simulink model "MIL_ASW"  (R2019b)
settings: Solver=FixedStepDiscrete  StartTime=0.0  StopTime=2  FixedStep=0.001  RelTol=1e-3  EnableMultiTasking=on
model workspace (MAT data in the model file):
  AccPedlCanVal : Simulink.Signal (value not decoded)
  AccPedlVal : Simulink.Signal (value not decoded)
  BrkPedlCanVal : Simulink.Signal (value not decoded)
  BrkPedlVal : Simulink.Signal (value not decoded)
  Cal1 : Simulink.Parameter (value not decoded)
  Cal10 : Simulink.Parameter (value not decoded)
  Cal11 : Simulink.Parameter (value not decoded)
  Cal12 : Simulink.Parameter (value not decoded)
  Cal2 : Simulink.Parameter (value not decoded)
  Cal3 : Simulink.Parameter (value not decoded)
  Cal4 : Simulink.Parameter (value not decoded)
  Cal5 : Simulink.Parameter (value not decoded)
  Cal6 : Simulink.Parameter (value not decoded)
  Cal7 : Simulink.Parameter (value not decoded)
  Cal8 : Simulink.Parameter (value not decoded)
  Cal9 : Simulink.Parameter (value not decoded)
  Clu1Act : Simulink.Signal (value not decoded)
  Clu1PTar : Simulink.Signal (value not decoded)
  Clu1Req : Simulink.Signal (value not decoded)
  Clu1TqTar : Simulink.Signal (value not decoded)
  Clu2Act : Simulink.Signal (value not decoded)
  Clu2PTar : Simulink.Signal (value not decoded)
  Clu2Req : Simulink.Signal (value not decoded)
  Clu2TqTar : Simulink.Signal (value not decoded)
  CluKissPtPLnch : Simulink.Parameter (value not decoded)
  CluOilTRawVal : Simulink.Signal (value not decoded)
  CluOilTVal : Simulink.Signal (value not decoded)
  CluOpenTqRatMax : Simulink.Parameter (value not decoded)
  CluPMap : Simulink.Parameter (value not decoded)
  CluPMax : Simulink.Parameter (value not decoded)
  CluPMaxGear1 : Simulink.Parameter (value not decoded)
  CluPMaxGear2 : Simulink.Parameter (value not decoded)
  CluPMaxGear3 : Simulink.Parameter (value not decoded)
  CluPMaxGear4 : Simulink.Parameter (value not decoded)
  CluPMaxGear5 : Simulink.Parameter (value not decoded)
  CluPMaxGear6 : Simulink.Parameter (value not decoded)
  CluPMaxGearR : Simulink.Parameter (value not decoded)
  CluPMin : Simulink.Parameter (value not decoded)
  CluPosnMax : Simulink.Parameter (value not decoded)
  CluSoln1IRawVal : Simulink.Signal (value not decoded)
  CluSoln1IReq : Simulink.Signal (value not decoded)
  CluSoln1IReqFlg : Simulink.Signal (value not decoded)
  CluSoln1IVal : Simulink.Signal (value not decoded)
  CluSoln1LineI : Simulink.Parameter (value not decoded)
  CluSoln1LineP : Simulink.Parameter (value not decoded)
  CluSoln1Pwm : Simulink.Signal (value not decoded)
  CluSoln2IRawVal : Simulink.Signal (value not decoded)
  CluSoln2IReq : Simulink.Signal (value not decoded)
  CluSoln2IReqFlg : Simulink.Signal (value not decoded)
  CluSoln2IVal : Simulink.Signal (value not decoded)
  CluSoln2LineI : Simulink.Parameter (value not decoded)
  CluSoln2LineP : Simulink.Parameter (value not decoded)
  CluSoln2Pwm : Simulink.Signal (value not decoded)
  CluTqMap : Simulink.Parameter (value not decoded)
  CrnkSpdRawVal : Simulink.Signal (value not decoded)
  CrnkSpdVal : Simulink.Signal (value not decoded)
  Drive_Intensity_Fuzzy : object (value not decoded)
  DrvIntenFzzy : Simulink.LookupTable (value not decoded)
  EngNIdle : Simulink.Parameter (value not decoded)
  EngNIdleMin : Simulink.Parameter (value not decoded)
  EngSpdCanVal : Simulink.Signal (value not decoded)
  EngThrCanVal : Simulink.Signal (value not decoded)
  EngTqAdd : Simulink.Parameter (value not decoded)
  EngTqCanVal : Simulink.Signal (value not decoded)
  EngTqIntvFlg : Simulink.Signal (value not decoded)
  EngTqIntvRat : Simulink.Signal (value not decoded)
  EngTqMapExtChartc : Simulink.Parameter (value not decoded)
  EngTqMapSpdIndx : Simulink.Parameter (value not decoded)
  EngTqMapThrtIndx : Simulink.Parameter (value not decoded)
  EngTqMapTqMax : Simulink.Parameter (value not decoded)
  EngTqMaxNorm : Simulink.Parameter (value not decoded)
  EngTqRef : Simulink.Parameter (value not decoded)
  EvenCluPRawVal : Simulink.Signal (value not decoded)
  EvenCluPVal : Simulink.Signal (value not decoded)
  EvenInpSpdRawVal : Simulink.Signal (value not decoded)
  EvenInpSpdVal : Simulink.Signal (value not decoded)
  FcnCallTime : Simulink.Parameter (value not decoded)
  FinalRat : Simulink.Parameter (value not decoded)
  Fork1A : Simulink.Parameter (value not decoded)
  Fork1Act : Simulink.Signal (value not decoded)
  Fork1B : Simulink.Parameter (value not decoded)
  Fork1DeltaSpdTar : Simulink.Parameter (value not decoded)
  Fork1MaxSpd1A : Simulink.Parameter (value not decoded)
  Fork1MaxSpd1B : Simulink.Parameter (value not decoded)
  Fork1MaxSpd2A : Simulink.Parameter (value not decoded)
  Fork1MaxSpd2B : Simulink.Parameter (value not decoded)
  Fork1PosnA : Simulink.Parameter (value not decoded)
  Fork1PosnB : Simulink.Parameter (value not decoded)
  Fork1PosnMaxSpd1A : Simulink.Parameter (value not decoded)
  Fork1PosnMaxSpd1B : Simulink.Parameter (value not decoded)
  Fork1PosnMaxSpd2A : Simulink.Parameter (value not decoded)
  Fork1PosnMaxSpd2B : Simulink.Parameter (value not decoded)
  Fork1PosnNeut : Simulink.Parameter (value not decoded)
  Fork1PosnNeutA : Simulink.Parameter (value not decoded)
  Fork1PosnNeutB : Simulink.Parameter (value not decoded)
  Fork1PosnRawVal : Simulink.Signal (value not decoded)
  Fork1PosnSyncA : Simulink.Parameter (value not decoded)
  Fork1PosnSyncB : Simulink.Parameter (value not decoded)
  Fork1PosnVal : Simulink.Signal (value not decoded)
  Fork1SyncTar : Simulink.Parameter (value not decoded)
  Fork2A : Simulink.Parameter (value not decoded)
  Fork2Act : Simulink.Signal (value not decoded)
  Fork2B : Simulink.Parameter (value not decoded)
  Fork2DeltaSpdTar : Simulink.Parameter (value not decoded)
  Fork2MaxSpd1A : Simulink.Parameter (value not decoded)
  Fork2MaxSpd1B : Simulink.Parameter (value not decoded)
  Fork2MaxSpd2A : Simulink.Parameter (value not decoded)
  Fork2MaxSpd2B : Simulink.Parameter (value not decoded)
  Fork2PosnA : Simulink.Parameter (value not decoded)
  Fork2PosnB : Simulink.Parameter (value not decoded)
  Fork2PosnMaxSpd1A : Simulink.Parameter (value not decoded)
  Fork2PosnMaxSpd1B : Simulink.Parameter (value not decoded)
  Fork2PosnMaxSpd2A : Simulink.Parameter (value not decoded)
  Fork2PosnMaxSpd2B : Simulink.Parameter (value not decoded)
  Fork2PosnNeut : Simulink.Parameter (value not decoded)
  Fork2PosnNeutA : Simulink.Parameter (value not decoded)
  Fork2PosnNeutB : Simulink.Parameter (value not decoded)
  Fork2PosnRawVal : Simulink.Signal (value not decoded)
  Fork2PosnSyncA : Simulink.Parameter (value not decoded)
  Fork2PosnSyncB : Simulink.Parameter (value not decoded)
  Fork2PosnVal : Simulink.Signal (value not decoded)
  Fork2SyncTar : Simulink.Parameter (value not decoded)
  Fork3A : Simulink.Parameter (value not decoded)
  Fork3Act : Simulink.Signal (value not decoded)
  Fork3B : Simulink.Parameter (value not decoded)
  Fork3DeltaSpdTar : Simulink.Parameter (value not decoded)
  Fork3MaxSpd1A : Simulink.Parameter (value not decoded)
  Fork3MaxSpd1B : Simulink.Parameter (value not decoded)
  Fork3MaxSpd2A : Simulink.Parameter (value not decoded)
  Fork3MaxSpd2B : Simulink.Parameter (value not decoded)
  Fork3PosnA : Simulink.Parameter (value not decoded)
  Fork3PosnB : Simulink.Parameter (value not decoded)
  Fork3PosnMaxSpd1A : Simulink.Parameter (value not decoded)
  Fork3PosnMaxSpd1B : Simulink.Parameter (value not decoded)
  Fork3PosnMaxSpd2A : Simulink.Parameter (value not decoded)
  Fork3PosnMaxSpd2B : Simulink.Parameter (value not decoded)
  Fork3PosnNeut : Simulink.Parameter (value not decoded)
  Fork3PosnNeutA : Simulink.Parameter (value not decoded)
  Fork3PosnNeutB : Simulink.Parameter (value not decoded)
  Fork3PosnRawVal : Simulink.Signal (value not decoded)
  Fork3PosnSyncA : Simulink.Parameter (value not decoded)
  Fork3PosnSyncB : Simulink.Parameter (value not decoded)
  Fork3PosnVal : Simulink.Signal (value not decoded)
  Fork3SyncTar : Simulink.Parameter (value not decoded)
  Fork4A : Simulink.Parameter (value not decoded)
  Fork4Act : Simulink.Signal (value not decoded)
  Fork4B : Simulink.Parameter (value not decoded)
  Fork4DeltaSpdTar : Simulink.Parameter (value not decoded)
  Fork4MaxSpd1A : Simulink.Parameter (value not decoded)
  Fork4MaxSpd1B : Simulink.Parameter (value not decoded)
  Fork4MaxSpd2A : Simulink.Parameter (value not decoded)
  Fork4MaxSpd2B : Simulink.Parameter (value not decoded)
  Fork4PosnA : Simulink.Parameter (value not decoded)
  Fork4PosnB : Simulink.Parameter (value not decoded)
  Fork4PosnMaxSpd1A : Simulink.Parameter (value not decoded)
  Fork4PosnMaxSpd1B : Simulink.Parameter (value not decoded)
  Fork4PosnMaxSpd2A : Simulink.Parameter (value not decoded)
  Fork4PosnMaxSpd2B : Simulink.Parameter (value not decoded)
  Fork4PosnNeut : Simulink.Parameter (value not decoded)
  Fork4PosnNeutA : Simulink.Parameter (value not decoded)
  Fork4PosnNeutB : Simulink.Parameter (value not decoded)
  Fork4PosnRawVal : Simulink.Signal (value not decoded)
  Fork4PosnSyncA : Simulink.Parameter (value not decoded)
  Fork4PosnSyncB : Simulink.Parameter (value not decoded)
  Fork4PosnVal : Simulink.Signal (value not decoded)
  Fork4SyncTar : Simulink.Parameter (value not decoded)
  FrntWhlRd : Simulink.Parameter (value not decoded)
  GearIdx : Simulink.Parameter (value not decoded)
  GearMax : Simulink.Parameter (value not decoded)
  GearRat : Simulink.Parameter (value not decoded)
  Launch_Engage_Fuzzy : object (value not decoded)
  LnchEngmtFzzy : Simulink.LookupTable (value not decoded)
  LubeSolnIRawVal : Simulink.Signal (value not decoded)
  LubeSolnIReq : Simulink.Signal (value not decoded)
  LubeSolnIVal : Simulink.Signal (value not decoded)
  LubeSolnLineI : Simulink.Parameter (value not decoded)
  LubeSolnLineP : Simulink.Parameter (value not decoded)
  LubeSolnPwm : Simulink.Signal (value not decoded)
  MaiLineSolnIRawVal : Simulink.Signal (value not decoded)
  MaiLineSolnIReq : Simulink.Signal (value not decoded)
  MaiLineSolnIVal : Simulink.Signal (value not decoded)
  MaiLineSolnLineI : Simulink.Parameter (value not decoded)
  MaiLineSolnLineP : Simulink.Parameter (value not decoded)
  MaiLineSolnPwm : Simulink.Signal (value not decoded)
  OddCluPRawVal : Simulink.Signal (value not decoded)
  OddCluPVal : Simulink.Signal (value not decoded)
  OddInpSpdRawVal : Simulink.Signal (value not decoded)
  OddInpSpdVal : Simulink.Signal (value not decoded)
  OutpSpdRawVal : Simulink.Signal (value not decoded)
  OutpSpdVal : Simulink.Signal (value not decoded)
  PsnsrLineP : Simulink.Parameter (value not decoded)
  PsnsrLineV : Simulink.Parameter (value not decoded)
  SftLvrCanVal : Simulink.Signal (value not decoded)
  SftLvrCfm : Simulink.Signal (value not decoded)
  SftLvrVal : Simulink.Signal (value not decoded)
  Shaft1GearAct : Simulink.Signal (value not decoded)
  Shaft1GearReq : Simulink.Signal (value not decoded)
  Shaft2GearAct : Simulink.Signal (value not decoded)
  Shaft2GearReq : Simulink.Signal (value not decoded)
  ShiftMux1SwtReq : Simulink.Signal (value not decoded)
  ShiftMux2SwtReq : Simulink.Signal (value not decoded)
  ShiftSdlEcoDwnSeln : Simulink.Parameter (value not decoded)
  ShiftSdlEcoDwnShift : Simulink.Parameter (value not decoded)
  ShiftSdlEcoUpSeln : Simulink.Parameter (value not decoded)
  ShiftSdlEcoUpShift : Simulink.Parameter (value not decoded)
  ShiftSdlPwrDwnSeln : Simulink.Parameter (value not decoded)
  ShiftSdlPwrDwnShift : Simulink.Parameter (value not decoded)
  ShiftSdlPwrUpSeln : Simulink.Parameter (value not decoded)
  ShiftSdlPwrUpShift : Simulink.Parameter (value not decoded)
  ShiftSdlSACDwnSeln : Simulink.Parameter (value not decoded)
  ShiftSdlSACDwnShift : Simulink.Parameter (value not decoded)
  ShiftSdlSACUpSeln : Simulink.Parameter (value not decoded)
  ShiftSdlSACUpShift : Simulink.Parameter (value not decoded)
  ShiftSdlThrPedlIdx : Simulink.Parameter (value not decoded)
  ShiftSoln1IRawVal : Simulink.Signal (value not decoded)
  ShiftSoln1IReq : Simulink.Signal (value not decoded)
  ShiftSoln1IVal : Simulink.Signal (value not decoded)
  ShiftSoln1LineI : Simulink.Parameter (value not decoded)
  ShiftSoln1LineP : Simulink.Parameter (value not decoded)
  ShiftSoln1Pwm : Simulink.Signal (value not decoded)
  ShiftSoln2IRawVal : Simulink.Signal (value not decoded)
  ShiftSoln2IReq : Simulink.Signal (value not decoded)
  ShiftSoln2IVal : Simulink.Signal (value not decoded)
  ShiftSoln2LineI : Simulink.Parameter (value not decoded)
  ShiftSoln2LineP : Simulink.Parameter (value not decoded)
  ShiftSoln2Pwm : Simulink.Signal (value not decoded)
  SolnOutpTRawVal : Simulink.Signal (value not decoded)
  SolnOutpTVal : Simulink.Signal (value not decoded)
  TSnsr1LineR : Simulink.Parameter (value not decoded)
  TSnsr2LineR : Simulink.Parameter (value not decoded)
  TrsmNrGearAct : Simulink.Signal (value not decoded)
  TrsmNrGearReq : Simulink.Signal (value not decoded)
  TrsmNrPreGearAct : Simulink.Signal (value not decoded)
  TrsmNrPreGearReq : Simulink.Signal (value not decoded)
  Tsnsr1LineT : Simulink.Parameter (value not decoded)
  Tsnsr2LineT : Simulink.Parameter (value not decoded)
  VehSpdCanVal : Simulink.Signal (value not decoded)
  VehSpdTrsmEstimd : Simulink.Signal (value not decoded)
  VehSpdVal : Simulink.Signal (value not decoded)
  VlvBodyTRawVal : Simulink.Signal (value not decoded)
  VlvBodyTVal : Simulink.Signal (value not decoded)
symbols that are objects in the model workspace (value not decoded): CluPMap, CluSoln1LineI, CluSoln1LineP, CluSoln2LineI, CluSoln2LineP, CluTqMap, EngNIdle, EngNIdleMin, EngTqMapThrtIndx, EngTqMapTqMax, EngTqMaxNorm, FcnCallTime, FinalRat, Fork1A, Fork1B, Fork1DeltaSpdTar, Fork1PosnA, Fork1PosnB, Fork1PosnMaxSpd1A, Fork1PosnMaxSpd1B, Fork1PosnMaxSpd2A, Fork1PosnMaxSpd2B, Fork1PosnNeut, Fork1PosnNeutA, Fork1PosnNeutB, Fork1PosnSyncA, Fork1PosnSyncB, Fork1SyncTar, Fork2A, Fork2B, Fork2DeltaSpdTar, Fork2PosnA, Fork2PosnB, Fork2PosnMaxSpd1A, Fork2PosnMaxSpd1B, Fork2PosnMaxSpd2A, Fork2PosnMaxSpd2B, Fork2PosnNeut, Fork2PosnNeutA, Fork2PosnNeutB, Fork2PosnSyncA, Fork2PosnSyncB, Fork2SyncTar, Fork3A, Fork3B, Fork3DeltaSpdTar, Fork3PosnA, Fork3PosnB, Fork3PosnMaxSpd1A, Fork3PosnMaxSpd1B, Fork3PosnMaxSpd2A, Fork3PosnMaxSpd2B, Fork3PosnNeut, Fork3PosnNeutA, Fork3PosnNeutB, Fork3PosnSyncA, Fork3PosnSyncB, Fork3SyncTar, Fork4A, Fork4B
undefined symbols (not defined in the file or in its folder): in1, out1
libraries: simulink x44, fuzblock x3
(part 2 of 10)

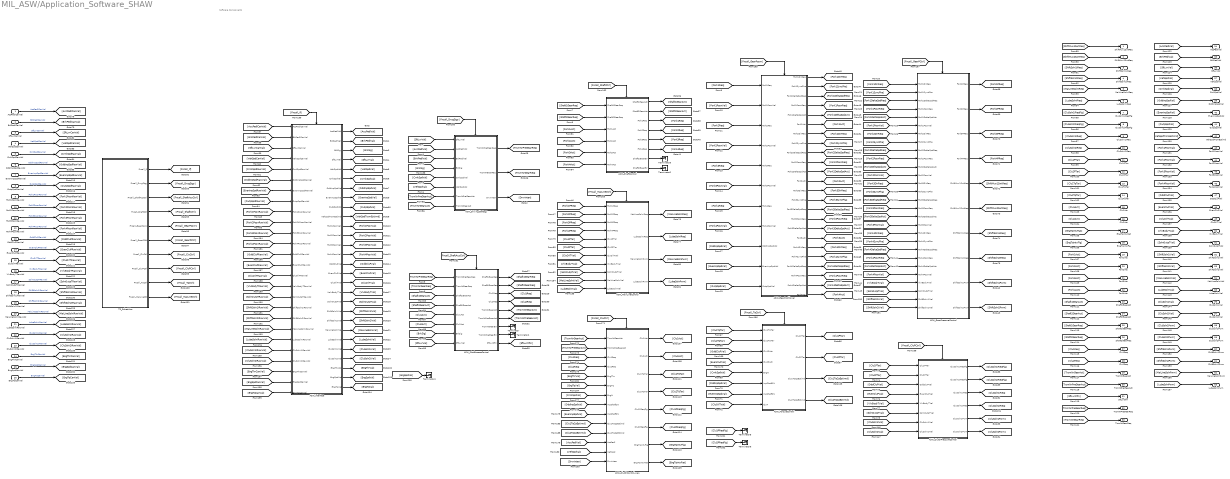
== system MIL_ASW/Application_Software_SHAW ==
  note: Software Components
  AccPedlCanVal : Inport
  BrkPedlCanVal : Inport  Port=2
  SftLvrCanVal : Inport  Port=3
  VehSpdCanVal : Inport  Port=4
  CrnkSpdRawVal : Inport  Port=5
  OddInpSpdRawVal : Inport  Port=6
  EvenInpSpdRawVal : Inport  Port=7
  OutpSpdRawVal : Inport  Port=8
  Fork1PosnRawVal : Inport  Port=9
  Fork2PosnRawVal : Inport  Port=10
  Fork3PosnRawVal : Inport  Port=11
  Fork4PosnRawVal : Inport  Port=12
  OddCluPRawVal : Inport  Port=13
  EvenCluPRawVal : Inport  Port=14
  CluOilTRawVal : Inport  Port=15
  VlvBodyTRawVal : Inport  Port=16
  SolnOutpTRawVal : Inport  Port=17
  ShiftSoln1IRawVal : Inport  Port=18
  ShiftSoln2IRawVal : Inport  Port=19
  MaiLineSolnIRawVal : Inport  Port=20
  LubeSolnIRawVal : Inport  Port=21
  CluSoln1IRawVal : Inport  Port=22
  CluSoln2IRawVal : Inport  Port=23
  EngThrCanVal : Inport  Port=24
  EngSpdCanVal : Inport  Port=25
  EngTqCanVal : Inport  Port=26
  ASW_ClutchControl_new : Subsystem  TreatAsAtomicUnit=on
  ASW_ClutchPressureControl : Subsystem  TreatAsAtomicUnit=on
  ASW_DrivingStrategy : Subsystem  TreatAsAtomicUnit=on
  ASW_GearPositioner : Subsystem
  ASW_GearPressureControl : Subsystem
  ASW_Interface : Subsystem
  ASW_MainLineControl : Subsystem  TreatAsAtomicUnit=on
  ASW_ShaftAccessControl : Subsystem
  ASW_ShaftControl : Subsystem
  ASW_TorqueControl : Subsystem  TreatAsAtomicUnit=on
  TR_Scheduler : Subsystem
  Terminator{,1..6} (7 alike) : Terminator
  ShiftMux1SwtReq : Outport  VectorParamsAs1DForOutWhenUnconnected=off
  ShiftMux2SwtReq : Outport  Port=2  VectorParamsAs1DForOutWhenUnconnected=off
  ShiftSoln1IReq : Outport  Port=3  VectorParamsAs1DForOutWhenUnconnected=off
  ShiftSoln2IReq : Outport  Port=4  VectorParamsAs1DForOutWhenUnconnected=off
  MaiLineSolnIReq : Outport  Port=5  VectorParamsAs1DForOutWhenUnconnected=off
  LubeSolnIReq : Outport  Port=6  VectorParamsAs1DForOutWhenUnconnected=off
  CluSoln1IReqFlg : Outport  Port=7  VectorParamsAs1DForOutWhenUnconnected=off
  CluSoln2IReqFlg : Outport  Port=8  VectorParamsAs1DForOutWhenUnconnected=off
  CluSoln1IReq : Outport  Port=9  VectorParamsAs1DForOutWhenUnconnected=off
  CluSoln2IReq : Outport  Port=10  VectorParamsAs1DForOutWhenUnconnected=off
  Clu1PTar : Outport  Port=11  OutDataTypeStr=uint16  VectorParamsAs1DForOutWhenUnconnected=off
  Clu2PTar : Outport  Port=12  OutDataTypeStr=uint16  VectorParamsAs1DForOutWhenUnconnected=off
  Clu1TqTar : Outport  Port=13  VectorParamsAs1DForOutWhenUnconnected=off
  Clu2TqTar : Outport  Port=14  VectorParamsAs1DForOutWhenUnconnected=off
  Clu1Act : Outport  Port=15  VectorParamsAs1DForOutWhenUnconnected=off
  Clu2Act : Outport  Port=16  VectorParamsAs1DForOutWhenUnconnected=off
  EngTqIntvRat : Outport  Port=17  VectorParamsAs1DForOutWhenUnconnected=off
  EngTqIntvFlg : Outport  Port=18  VectorParamsAs1DForOutWhenUnconnected=off
  Fork1Act : Outport  Port=19  VectorParamsAs1DForOutWhenUnconnected=off
  Fork2Act : Outport  Port=20  VectorParamsAs1DForOutWhenUnconnected=off
  Fork3Act : Outport  Port=21  VectorParamsAs1DForOutWhenUnconnected=off
  Fork4Act : Outport  Port=22  VectorParamsAs1DForOutWhenUnconnected=off
  Shaft1GearAct : Outport  Port=23  VectorParamsAs1DForOutWhenUnconnected=off
  Shaft2GearAct : Outport  Port=24  VectorParamsAs1DForOutWhenUnconnected=off
  Shaft1GearReq : Outport  Port=25  VectorParamsAs1DForOutWhenUnconnected=off
  Shaft2GearReq : Outport  Port=26  VectorParamsAs1DForOutWhenUnconnected=off
  Clu1Req : Outport  Port=27  VectorParamsAs1DForOutWhenUnconnected=off
  Clu2Req : Outport  Port=28  VectorParamsAs1DForOutWhenUnconnected=off
  TrsmNrGearAct : Outport  Port=29  VectorParamsAs1DForOutWhenUnconnected=off
  TrsmNrPreGearAct : Outport  Port=30  VectorParamsAs1DForOutWhenUnconnected=off
  SftLvrCfm : Outport  Port=31  VectorParamsAs1DForOutWhenUnconnected=off
  TrsmNrPreGearReq : Outport  Port=32  OutDataTypeStr=uint8  VectorParamsAs1DForOutWhenUnconnected=off
  TrsmNrGearReq : Outport  Port=33  OutDataTypeStr=uint8  VectorParamsAs1DForOutWhenUnconnected=off
  AccPedlVal : Outport  Port=34  VectorParamsAs1DForOutWhenUnconnected=off
  BrkPedlVal : Outport  Port=35  OutDataTypeStr=uint8  VectorParamsAs1DForOutWhenUnconnected=off
  SftLvrVal : Outport  Port=36  OutDataTypeStr=uint8  VectorParamsAs1DForOutWhenUnconnected=off
  VehSpdVal : Outport  Port=37  VectorParamsAs1DForOutWhenUnconnected=off
  CrnkSpdVal : Outport  Port=38  VectorParamsAs1DForOutWhenUnconnected=off
  OddInpSpdVal : Outport  Port=39  VectorParamsAs1DForOutWhenUnconnected=off
  EvenInpSpdVal : Outport  Port=40  VectorParamsAs1DForOutWhenUnconnected=off
  OutpSpdVal : Outport  Port=41  VectorParamsAs1DForOutWhenUnconnected=off
  VehSpdTrsmEstimd : Outport  Port=42  VectorParamsAs1DForOutWhenUnconnected=off
  Fork1PosnVal : Outport  Port=43  VectorParamsAs1DForOutWhenUnconnected=off
  Fork2PosnVal : Outport  Port=44  VectorParamsAs1DForOutWhenUnconnected=off
  Fork3PosnVal : Outport  Port=45  VectorParamsAs1DForOutWhenUnconnected=off
  Fork4PosnVal : Outport  Port=46  VectorParamsAs1DForOutWhenUnconnected=off
  OddCluPVal : Outport  Port=47  VectorParamsAs1DForOutWhenUnconnected=off
  EvenCluPVal : Outport  Port=48  VectorParamsAs1DForOutWhenUnconnected=off
  CluOilTVal : Outport  Port=49  VectorParamsAs1DForOutWhenUnconnected=off
  VlvBodyTVal : Outport  Port=50  VectorParamsAs1DForOutWhenUnconnected=off
  SolnOutpTVal : Outport  Port=51  VectorParamsAs1DForOutWhenUnconnected=off
  ShiftSoln1IVal : Outport  Port=52  VectorParamsAs1DForOutWhenUnconnected=off
  ShiftSoln2IVal : Outport  Port=53  VectorParamsAs1DForOutWhenUnconnected=off
  MaiLineSolnIVal : Outport  Port=54  VectorParamsAs1DForOutWhenUnconnected=off
  LubeSolnIVal : Outport  Port=55  VectorParamsAs1DForOutWhenUnconnected=off
  CluSoln1IVal : Outport  Port=56  VectorParamsAs1DForOutWhenUnconnected=off
  CluSoln2IVal : Outport  Port=57  VectorParamsAs1DForOutWhenUnconnected=off
  CluSoln1Pwm : Outport  Port=58  VectorParamsAs1DForOutWhenUnconnected=off
  CluSoln2Pwm : Outport  Port=59  VectorParamsAs1DForOutWhenUnconnected=off
  ShiftSoln1Pwm : Outport  Port=60  VectorParamsAs1DForOutWhenUnconnected=off
  ShiftSoln2Pwm : Outport  Port=61  VectorParamsAs1DForOutWhenUnconnected=off
  MaiLineSolnPwm : Outport  Port=62  VectorParamsAs1DForOutWhenUnconnected=off
  LubeSolnPwm : Outport  Port=63  VectorParamsAs1DForOutWhenUnconnected=off
  wires:
  [ShiftMux1SwtReq] -> ShiftMux1SwtReq/1
  [ShiftMux2SwtReq] -> ShiftMux2SwtReq/1
  [ShiftSoln1IReq] -> ShiftSoln1IReq/1
  [ShiftSoln2IReq] -> ShiftSoln2IReq/1
  [MaiLineSolnIReq] -> MaiLineSolnIReq/1
  [LubeSolnIReq] -> LubeSolnIReq/1
  [CluSoln1IReqFlg] -> CluSoln1IReqFlg/1
  [CluSoln2IReqFlg] -> CluSoln2IReqFlg/1
  [CluSoln1IReq] -> CluSoln1IReq/1
  [CluSoln2IReq] -> CluSoln2IReq/1
  [Clu1PTar] -> Clu1PTar/1
  [Clu2PTar] -> Clu2PTar/1
  [Clu1TqTar] -> Clu1TqTar/1
  [Clu2TqTar] -> Clu2TqTar/1
  [Clu1Act] -> Clu1Act/1
  [Clu2Act] -> Clu2Act/1
  [EngTqIntvRat] -> EngTqIntvRat/1
  [EngTqIntvFlg] -> EngTqIntvFlg/1
  [Fork1Act] -> Fork1Act/1
  [Fork2Act] -> Fork2Act/1
  [Fork3Act] -> Fork3Act/1
  [Fork4Act] -> Fork4Act/1
  [Shaft1GearAct] -> Shaft1GearAct/1
  [Shaft2GearAct] -> Shaft2GearAct/1
  [Shaft1GearReq] -> Shaft1GearReq/1
  [Shaft2GearReq] -> Shaft2GearReq/1
  [Clu1Req] -> Clu1Req/1
  [Clu2Req] -> Clu2Req/1
  [TrsmNrGearAct] -> TrsmNrGearAct/1
  [TrsmNrPreGearAct] -> TrsmNrPreGearAct/1
  [SftLvrCfm] -> SftLvrCfm/1
  [TrsmNrPreGearReq] -> TrsmNrPreGearReq/1
  [TrsmNrGearReq] -> TrsmNrGearReq/1
  [AccPedlVal] -> AccPedlVal/1
  [BrkPedlVal] -> BrkPedlVal/1
  [SftLvrVal] -> SftLvrVal/1
  [VehSpdVal] -> VehSpdVal/1
  [CrnkSpdVal] -> CrnkSpdVal/1
  [OddInpSpdVal] -> OddInpSpdVal/1
  [EvenInpSpdVal] -> EvenInpSpdVal/1
  [OutpSpdVal] -> OutpSpdVal/1
  [VehSpdTrsmEstimd] -> VehSpdTrsmEstimd/1
  [Fork1PosnVal] -> Fork1PosnVal/1
  [Fork2PosnVal] -> Fork2PosnVal/1
  [Fork3PosnVal] -> Fork3PosnVal/1
  [Fork4PosnVal] -> Fork4PosnVal/1
  [OddCluPVal] -> OddCluPVal/1
  [EvenCluPVal] -> EvenCluPVal/1
  [CluOilTVal] -> CluOilTVal/1
  [VlvBodyTVal] -> VlvBodyTVal/1
  [SolnOutpTVal] -> SolnOutpTVal/1
  [ShiftSoln1IVal] -> ShiftSoln1IVal/1
  [ShiftSoln2IVal] -> ShiftSoln2IVal/1
  [MaiLineSolnIVal] -> MaiLineSolnIVal/1
  [LubeSolnIVal] -> LubeSolnIVal/1
  [CluSoln1IVal] -> CluSoln1IVal/1
  [CluSoln2IVal] -> CluSoln2IVal/1
  [CluSoln1Pwm] -> CluSoln1Pwm/1
  [CluSoln2Pwm] -> CluSoln2Pwm/1
  [ShiftSoln1Pwm] -> ShiftSoln1Pwm/1
  [ShiftSoln2Pwm] -> ShiftSoln2Pwm/1
  [MaiLineSolnPwm] -> MaiLineSolnPwm/1
  [LubeSolnPwm] -> LubeSolnPwm/1
  TR_Scheduler/1(Fncall_If) -> [Fncall_If]
  TR_Scheduler/2(Fncall_DrvgStgy) -> [Fncall_DrvgStgy]
  TR_Scheduler/3(Fncall_ShaftAcsCtrl) -> [Fncall_ShaftAcsCtrl]
  TR_Scheduler/10(Fncall_MaiLineCtrl) -> [Fncall_MaiLineCtrl]
  TR_Scheduler/4(Fncall_ShaftCtrl) -> [Fncall_ShaftCtrl]
  TR_Scheduler/6(Fncall_GearPCtrl) -> [Fncall_GearPCtrl]
  TR_Scheduler/7(Fncall_CluCtrl) -> [Fncall_CluCtrl]
  TR_Scheduler/8(Fncall_CluPCtrl) -> [Fncall_CluPCtrl]
  TR_Scheduler/5(Fncall_GearPosnr) -> [Fncall_GearPosnr]
  TR_Scheduler/9(Fncall_TqCtrl) -> [Fncall_TqCtrl]
  AccPedlCanVal/1 -> [AccPedlCanVal]  "AccPedlCanVal"
  BrkPedlCanVal/1 -> [BrkPedlCanVal]  "BrkPedlCanVal"
  SftLvrCanVal/1 -> [SftLvrCanVal]  "SftLvrCanVal"
  VehSpdCanVal/1 -> [VehSpdCanVal]  "VehSpdCanVal"
  CrnkSpdRawVal/1 -> [CrnkSpdRawVal]  "CrnkSpdRawVal"
  OddInpSpdRawVal/1 -> [OddInpSpdRawVal]  "OddInpSpdRawVal"
  EvenInpSpdRawVal/1 -> [EvenInpSpdRawVal]  "EvenInpSpdRawVal"
  OutpSpdRawVal/1 -> [OutpSpdRawVal]  "OutpSpdRawVal"
  Fork1PosnRawVal/1 -> [Fork1PosnRawVal]  "Fork1PosnRawVal"
  Fork2PosnRawVal/1 -> [Fork2PosnRawVal]  "Fork2PosnRawVal"
  Fork3PosnRawVal/1 -> [Fork3PosnRawVal]  "Fork3PosnRawVal"
  Fork4PosnRawVal/1 -> [Fork4PosnRawVal]  "Fork4PosnRawVal"
  OddCluPRawVal/1 -> [OddCluPRawVal]  "OddCluPRawVal"
  EvenCluPRawVal/1 -> [EvenCluPRawVal]  "EvenCluPRawVal"
  CluOilTRawVal/1 -> [CluOilTRawVal]  "CluOilTRawVal"
  VlvBodyTRawVal/1 -> [VlvBodyTRawVal]  "VlvBodyTRawVal"
  SolnOutpTRawVal/1 -> [SolnOutpTRawVal]  "SolnOutpTRawVal"
  ShiftSoln1IRawVal/1 -> [ShiftSoln1IRawVal]  "ShiftSoln1IRawVal"
  ShiftSoln2IRawVal/1 -> [ShiftSoln2IRawVal]  "ShiftSoln2IRawVal"
  MaiLineSolnIRawVal/1 -> [MaiLineSolnIRawVal]  "MaiLineSolnIRawVal"
  LubeSolnIRawVal/1 -> [LubeSolnIRawVal]  "LubeSolnIRawVal"
  CluSoln1IRawVal/1 -> [CluSoln1IRawVal]  "CluSoln1IRawVal"
  CluSoln2IRawVal/1 -> [CluSoln2IRawVal]  "CluSoln2IRawVal"
  EngThrCanVal/1 -> [EngThrCanVal]  "EngThrCanVal"
  EngSpdCanVal/1 -> [EngSpdCanVal]  "EngSpdCanVal"
  EngTqCanVal/1 -> [EngTqCanVal]  "EngTqCanVal"
  ASW_GearPressureControl/10(ShiftSoln2Pwm) -> [ShiftSoln2Pwm]
  [Fncall_GearPCtrl] -> ASW_GearPressureControl/Trigger
  [CluSoln1IRawVal] -> ASW_Interface/22(CluSoln1IRawVal)
  ASW_GearPressureControl/8(ShiftSoln2IReq) -> [ShiftSoln2IReq]
  ASW_Interface/6(CrnkSpdVal) -> [CrnkSpdVal]
  ASW_GearPositioner/13(Fork3DirReq) -> [Fork3DirReq]
  [Clu2PReqFlg] -> Terminator6/1
  ASW_ClutchPressureControl/5(CluSoln1Pwm) -> [CluSoln1Pwm]
  [Fork4Req] -> ASW_GearPositioner/7(Fork4Req)
  ASW_GearPressureControl/5(ShiftMux1SwtReq) -> [ShiftMux1SwtReq]
  [Clu1TqCpEstimd] -> ASW_ClutchControl_new/10(Clu1TqCpEstimd)
  ASW_MainLineControl/3(MaiLineSolnPwm) -> [MaiLineSolnPwm]
  [AccPedlVal] -> ASW_DrivingStrategy/2(AccPedlVal)
  ASW_ClutchControl_new/3(Clu1TqTar) -> [Clu1TqTar]
  ASW_GearPositioner/4(Fork1PosnReq) -> [Fork1PosnReq]
  ASW_Interface/4(SftLvrVal) -> [SftLvrVal]
  ASW_GearPositioner/23(Fork4DeltaSpdAct) -> [Fork4DeltaSpdAct]
  ASW_Interface/7(OddInpSpdVal) -> [OddInpSpdVal]
  ASW_GearPositioner/8(Fork2SyncPha) -> [Fork2SyncPha]
  ASW_GearPressureControl/7(ShiftSoln1IReq) -> [ShiftSoln1IReq]
  [Fncall_CluPCtrl] -> ASW_ClutchPressureControl/Trigger
  [Fork2PReq] -> ASW_MainLineControl/2(Fork2PReq)
  ASW_Interface/17(CluOilTVal) -> [CluOilTVal]
  ASW_GearPositioner/18(Fork3Act) -> [Fork3Act]
  [OddInpSpdVal] -> ASW_ClutchControl_new/8(InpShaft1N)
  [CluOilTVal] -> ASW_MainLineControl/7(CluOilTVal)
  ASW_ShaftAccessControl/4(Clu2Req) -> [Clu2Req]
  [Fork1DeltaSpdReq] -> ASW_GearPressureControl/3(Fork1DeltaSpdReq)
  ASW_ShaftAccessControl/8(TrsmNrPreGearErr) -> Terminator1/1
  ASW_Interface/15(OddCluPVal) -> [OddCluPVal]
  ASW_TorqueControl/4(Clu2TqCpEstimd) -> [Clu2TqCpEstimd]
  [Clu2Req] -> ASW_ClutchControl_new/4(Clu2Req)
  [ShiftSoln2IVal] -> ASW_GearPressureControl/28(ShiftSoln2IVal)
  [Fork4PosnVal] -> ASW_GearPressureControl/24(Fork4PosnVal)
  [VehSpdVal] -> ASW_ClutchControl_new/13(VehSpd)
  [Fork4SyncPha] -> ASW_GearPressureControl/20(Fork4SyncPha)
  ASW_ClutchControl_new/5(Clu1PReqFlg) -> [Clu1PReqFlg]
  [Fork4PosnReq] -> ASW_GearPressureControl/22(Fork4PosnReq)
  [Fork1PosnVal] -> ASW_GearPressureControl/6(Fork1PosnVal)
  ASW_TorqueControl/2(Clu2PTar) -> [Clu2PTar]
  [Fork1SyncPha] -> ASW_GearPressureControl/2(Fork1SyncPha)
  [Fork4DeltaSpdReq] -> ASW_GearPressureControl/21(Fork4DeltaSpdReq)
  [EngThrVal] -> ASW_ClutchControl_new/5(EngThr)
  ASW_Interface/9(OutpSpdVal) -> [OutpSpdVal]
  [SolnOutpTVal] -> ASW_ClutchPressureControl/6(SolnOutpTVal)
  [Fork1PReq] -> ASW_MainLineControl/1(Fork1PReq)
  ASW_ShaftControl/3(Fork1Req) -> [Fork1Req]
  ASW_MainLineControl/4(LubeSolnPwm) -> [LubeSolnPwm]
  ASW_MainLineControl/2(LubeSolnIReq) -> [LubeSolnIReq]
  [Fork3PosnVal] -> ASW_GearPressureControl/18(Fork3PosnVal)
  [Fork1DeltaSpdAct] -> ASW_GearPressureControl/5(Fork1DeltaSpdAct)
  ASW_Interface/18(ValvBodyTVal) -> [VlvBodyTVal]
  [Fncall_CluCtrl] -> ASW_ClutchControl_new/Trigger
  [CrnkSpdVal] -> ASW_ClutchControl_new/7(EngN)
  [ShiftSoln1IVal] -> ASW_GearPressureControl/27(ShiftSoln1IVal)
  [OddCluPVal] -> ASW_TorqueControl/3(Clu1PAct)
  [Fork3PReq] -> ASW_MainLineControl/3(Fork3PReq)
  [CluSoln2IVal] -> ASW_ClutchPressureControl/8(CluSoln2IVal)
  [Fork1Act] -> ASW_ShaftControl/3(Fork1Act)
  [Clu2PTar] -> ASW_MainLineControl/6(Clu2PTar)
  ASW_GearPositioner/14(Fork3SyncPha) -> [Fork3SyncPha]
  ASW_GearPositioner/17(Fork3DeltaSpdAct) -> [Fork3DeltaSpdAct]
  [Fork3PosnReq] -> ASW_GearPressureControl/16(Fork3PosnReq)
  ASW_GearPositioner/16(Fork3PosnReq) -> [Fork3PosnReq]
  ASW_ClutchControl_new/7(EngTqIntvFlg) -> [EngTqIntvFlg]
  [TrsmNrGearReq] -> ASW_ShaftAccessControl/2("TrsmNrGearReq ")
  ASW_GearPositioner/12(Fork2Act) -> [Fork2Act]
  ASW_GearPressureControl/9(ShiftSoln1Pwm) -> [ShiftSoln1Pwm]
  [Fork2PosnVal] -> ASW_GearPressureControl/12(Fork2PosnVal)
  ASW_Interface/1(AccPedlVal) -> [AccPedlVal]
  ASW_GearPressureControl/2(Fork2PReq) -> [Fork2PReq]
  [EngTqCanVal] -> ASW_Interface/26(EngTqCanVal)
  [Fncall_DrvgStgy] -> ASW_DrivingStrategy/Trigger
  ASW_ClutchPressureControl/1(CluSoln1IReqFlg) -> [CluSoln1IReqFlg]
  ASW_ShaftAccessControl/3(Clu1Req) -> [Clu1Req]
  ASW_DrivingStrategy/1(TrsmNrPreGearReq) -> [TrsmNrPreGearReq]
  ASW_Interface/16(EvenCluPVal) -> [EvenCluPVal]
  ASW_GearPressureControl/6(ShiftMux2SwtReq) -> [ShiftMux2SwtReq]
  [Fork3Req] -> ASW_GearPositioner/5(Fork3Req)
  [EvenCluPRawVal] -> ASW_Interface/14(EvenCluPRawVal)
  [OddCluPRawVal] -> ASW_Interface/13(OddCluPRawVal)
  ASW_ShaftAccessControl/5(TrsmNrGearAct) -> [TrsmNrGearAct]
  ASW_Interface/23(LubeSolnIVal) -> [LubeSolnIVal]
  ASW_Interface/25(CluSoln2IVal) -> [CluSoln2IVal]
  ASW_GearPressureControl/1(Fork1PReq) -> [Fork1PReq]
  [Fork2Act] -> ASW_ShaftControl/4(Fork2Act)
  ASW_GearPositioner/5(Fork1DeltaSpdAct) -> [Fork1DeltaSpdAct]
  ASW_Interface/28(EngTqVal) -> [EngTqVal]
  ASW_DrivingStrategy/2(TrsmNrGearReq) -> [TrsmNrGearReq]
  ASW_ShaftAccessControl/6(TrsmNrPreGearAct) -> [TrsmNrPreGearAct]
  [ShiftSoln2IRawVal] -> ASW_Interface/19(ShiftSoln2IRawVal)
  [Fork3PosnRawVal] -> ASW_Interface/11(Fork3PosnRawVal)
  [SftLvrVal] -> ASW_DrivingStrategy/1(SftLvrVal)
  ASW_GearPositioner/1(Fork1DirReq) -> [Fork1DirReq]
  ASW_ClutchControl_new/4(Clu2TqTar) -> [Clu2TqTar]
  [Fork2DirReq] -> ASW_GearPressureControl/7(Fork2DirReq)
  [Fork2PosnVal] -> ASW_GearPositioner/4(Fork2PosnVal)
  ASW_Interface/11(Fork1PosnVal) -> [Fork1PosnVal]
  [Fork4DirReq] -> ASW_GearPressureControl/19(Fork4DirReq)
  [CrnkSpdVal] -> ASW_TorqueControl/5(EngN)
  [AccPedlVal] -> ASW_ClutchControl_new/12(AccPedl)
  ASW_Interface/26(EngThrVal) -> [EngThrVal]
  [MaiLineSolnIRawVal] -> ASW_Interface/20(MaiLineSolnIRawVal)
  ASW_Interface/13(Fork3PosnVal) -> [Fork3PosnVal]
  [VlvBodyTVal] -> ASW_GearPressureControl/25(VlvBodyTVal)
  [Fork4PReq] -> ASW_MainLineControl/4(Fork4PReq)
  ASW_Interface/8(EvenInpSpdVal) -> [EvenInpSpdVal]
  ASW_GearPositioner/21(Fork4DeltaSpdReq) -> [Fork4DeltaSpdReq]
  [Fncall_If] -> ASW_Interface/Trigger
  [Fncall_ShaftAcsCtrl] -> ASW_ShaftAccessControl/Trigger
  [TrsmNrGearAct] -> ASW_ClutchControl_new/1(TrsmNrGearAct)
  [SftLvrVal] -> ASW_ShaftAccessControl/8(SftLvrVal)
  [Clu1TqTar] -> ASW_TorqueControl/1(Clu1TqTar)
  [Fork3Act] -> ASW_ShaftControl/5(Fork3Act)
  ASW_ShaftAccessControl/9(SftLvrCfm) -> [SftLvrCfm]
  [Fork1DirReq] -> ASW_GearPressureControl/1(Fork1DirReq)
  [BrkPedlVal] -> ASW_DrivingStrategy/3(BrkPedlVal)
  [Fork3PosnVal] -> ASW_GearPositioner/6(Fork3PosnVal)
  ASW_GearPositioner/3(Fork1DeltaSpdReq) -> [Fork1DeltaSpdReq]
  ASW_GearPositioner/10(Fork2PosnReq) -> [Fork2PosnReq]
  [TrsmNrPreGearAct] -> ASW_DrivingStrategy/7(TrsmNrPreGearAct)
  [Clu2TqTar] -> ASW_TorqueControl/2(Clu2TqTar)
  [OutpSpdRawVal] -> ASW_Interface/8(OutpSpdRawVal)
  [Fork4Act] -> ASW_ShaftControl/6(Fork4Act)
  [VehSpdVal] -> ASW_DrivingStrategy/6(VehSpdVal)
  ASW_DrivingStrategy/3(DrvrInten) -> [DrvrInten]
  ASW_ShaftControl/1(Shaft1GearAct) -> [Shaft1GearAct]
  ASW_ClutchControl_new/8(EngTqIntvRat) -> [EngTqIntvRat]
  [Fncall_TqCtrl] -> ASW_TorqueControl/Trigger
  ASW_ShaftControl/6(Fork4Req) -> [Fork4Req]
  ASW_ClutchControl_new/6(Clu2PReqFlg) -> [Clu2PReqFlg]
  [Fork3DeltaSpdAct] -> ASW_GearPressureControl/17(Fork3DeltaSpdAct)
  [BrkPedlCanVal] -> ASW_Interface/2(BrkPedlCanVal)
  [Clu1PTar] -> ASW_ClutchPressureControl/1(Clu1PTar)
  [EvenInpSpdVal] -> ASW_TorqueControl/7(InpShaft2N)
  [Fork4PosnVal] -> ASW_GearPositioner/8(Fork4PosnVal)
  [LubeSolnIVal] -> ASW_MainLineControl/11(LubeSolnIVal)
  ASW_GearPositioner/2(Fork1SyncPha) -> [Fork1SyncPha]
  [SolnOutpTVal] -> ASW_MainLineControl/9(SolnOutpTVal)
  [CluOilTVal] -> ASW_TorqueControl/8(CluT)
  [SolnOutpTRawVal] -> ASW_Interface/17(SolnOutpTRawVal)
  ASW_GearPressureControl/3(Fork3PReq) -> [Fork3PReq]
  [Fork4PosnRawVal] -> ASW_Interface/12(Fork4PosnRawVal)
  ASW_TorqueControl/1(Clu1PTar) -> [Clu1PTar]
  [OddInpSpdRawVal] -> ASW_Interface/6(OddInpSpdRawVal)
  ASW_GearPositioner/11(Fork2DeltaSpdAct) -> [Fork2DeltaSpdAct]
  ASW_GearPositioner/15(Fork3DeltaSpdReq) -> [Fork3DeltaSpdReq]
  ASW_ShaftControl/5(Fork3Req) -> [Fork3Req]
  [DrvrInten] -> ASW_ClutchControl_new/14(DrvrInten)
  ASW_Interface/2(BrkPedlVal) -> [BrkPedlVal]
  [EngThrCanVal] -> ASW_Interface/24(EngThrCanVal)
  ASW_ShaftAccessControl/2(Shaft2GearReq) -> [Shaft2GearReq]
  [Clu1PTar] -> ASW_MainLineControl/5(Clu1PTar)
  [BrkSig] -> ASW_DrivingStrategy/4(BrkSig)
  ASW_ClutchControl_new/1(Clu1Act) -> [Clu1Act]
  [TrsmNrGearAct] -> ASW_DrivingStrategy/8(TrsmNrGearAct)
  [CrnkSpdRawVal] -> ASW_Interface/5(CrnkSpdRawVal)
  [Fork4DeltaSpdAct] -> ASW_GearPressureControl/23(Fork4DeltaSpdAct)
  ASW_Interface/24(CluSoln1IVal) -> [CluSoln1IVal]
  [Fork3SyncPha] -> ASW_GearPressureControl/14(Fork3SyncPha)
  [Fork2SyncPha] -> ASW_GearPressureControl/8(Fork2SyncPha)
  [Fncall_GearPosnr] -> ASW_GearPositioner/Trigger
  ASW_GearPositioner/20(Fork4SyncPha) -> [Fork4SyncPha]
  [Fork1PosnRawVal] -> ASW_Interface/9(Fork1PosnRawVal)
  ASW_TorqueControl/3(Clu1TqCpEstimd) -> [Clu1TqCpEstimd]
  ASW_Interface/14(Fork4PosnVal) -> [Fork4PosnVal]
  [Clu2TqCpEstimd] -> ASW_ClutchControl_new/11(Clu2TqCpEstimd)
  [EvenCluPVal] -> ASW_TorqueControl/4(Clu2PAct)
  [Clu2Act] -> ASW_ShaftAccessControl/6("Clu2Act ")
  [VlvBodyTRawVal] -> ASW_Interface/16(ValvBodyTRawVal)
  [Fork2DeltaSpdReq] -> ASW_GearPressureControl/9(Fork2DeltaSpdReq)
  ASW_GearPositioner/9(Fork2DeltaSpdReq) -> [Fork2DeltaSpdReq]
  ASW_Interface/20(ShiftSoln1IVal) -> [ShiftSoln1IVal]
  [EvenInpSpdVal] -> ASW_GearPositioner/10(EvenInpSpdVal)
  [Fork2Req] -> ASW_GearPositioner/3(Fork2Req)
  [EvenInpSpdVal] -> ASW_ClutchControl_new/9(InpShaft2N)
  [Clu1Act] -> ASW_ShaftAccessControl/5("Clu1Act ")
  [Shaft1GearAct] -> ASW_ShaftAccessControl/3("Shaft1GearAct ")
  [LubeSolnIRawVal] -> ASW_Interface/21(LubeSolnIRawVal)
  [EvenInpSpdRawVal] -> ASW_Interface/7(EvenInpSpdRawVal)
  ASW_GearPositioner/22(Fork4PosnReq) -> [Fork4PosnReq]
  ASW_ShaftAccessControl/1(Shaft1GearReq) -> [Shaft1GearReq]
  [Fork1PosnVal] -> ASW_GearPositioner/2(Fork1PosnVal)
  [OddCluPVal] -> ASW_ClutchPressureControl/3(OddCluPVal)
  ASW_ClutchPressureControl/6(CluSoln2Pwm) -> [CluSoln2Pwm]
  ASW_GearPositioner/6(Fork1Act) -> [Fork1Act]
  [OddInpSpdVal] -> ASW_TorqueControl/6(InpShaft1N)
  [CluOilTRawVal] -> ASW_Interface/15(CluOilTRawVal)
  ASW_ShaftControl/2(Shaft2GearAct) -> [Shaft2GearAct]
  [Fork1Req] -> ASW_GearPositioner/1(Fork1Req)
  [Clu2PTar] -> ASW_ClutchPressureControl/2(Clu2PTar)
  ASW_ClutchPressureControl/3(CluSoln1IReq) -> [CluSoln1IReq]
  [VlvBodyTVal] -> ASW_ClutchPressureControl/5(VlvBodyTVal)
  [EvenCluPVal] -> ASW_ClutchPressureControl/4(EvenCluPVal)
  [CluSoln1IVal] -> ASW_ClutchPressureControl/7(CluSoln1IVal)
  ASW_Interface/19(SolnOutpTVal) -> [SolnOutpTVal]
  [Fork3DirReq] -> ASW_GearPressureControl/13(Fork3DirReq)
  [OutpSpdVal] -> ASW_GearPositioner/11(OutpSpdVal)
  [Clu1Req] -> ASW_ClutchControl_new/3(Clu1Req)
  [MaiLineSolnIVal] -> ASW_MainLineControl/10(MaiLineSolnIVal)
  [BrkSig] -> ASW_ShaftAccessControl/7(BrkSig)
  ASW_ShaftControl/4(Fork2Req) -> [Fork2Req]
  ASW_ShaftControl/8(Shaft2GearErr) -> Terminator2/1
  ASW_GearPositioner/24(Fork4Act) -> [Fork4Act]
  [TrsmNrPreGearAct] -> ASW_ClutchControl_new/2(TrsmNrPreGearAct)
  ASW_GearPressureControl/4(Fork4PReq) -> [Fork4PReq]
  [Fork2PosnRawVal] -> ASW_Interface/10(Fork24PosnRawVal)
  ASW_MainLineControl/1(MaiLineSolnIReq) -> [MaiLineSolnIReq]
  ASW_ClutchPressureControl/2(CluSoln2IReqFlg) -> [CluSoln2IReqFlg]
  [OddInpSpdVal] -> ASW_GearPositioner/9(OddInpSpdVal)
  ASW_Interface/3(BrkSig) -> [BrkSig]
  ASW_Interface/21(ShiftSoln2IVal) -> [ShiftSoln2IVal]
  [Fork2PosnReq] -> ASW_GearPressureControl/10(Fork2PosnReq)
  [CrnkSpdVal] -> ASW_DrivingStrategy/5(CrnkSpdVal)
  [SftLvrCanVal] -> ASW_Interface/3(SftLvrCanVal)
  ASW_GearPositioner/7(Fork2DirReq) -> [Fork2DirReq]
  [TrsmNrPreGearReq] -> ASW_ShaftAccessControl/1("TrsmNrPreGearReq ")
  [VlvBodyTVal] -> ASW_MainLineControl/8(VlvBodyTVal)
  ASW_Interface/27(EngSpdVal) -> [EngSpdVal]
  [Fncall_MaiLineCtrl] -> ASW_MainLineControl/Trigger
  ASW_Interface/5(VehSpdVal) -> [VehSpdVal]
  [ShiftSoln1IRawVal] -> ASW_Interface/18(ShiftSoln1IRawVal)
  [Shaft1GearReq] -> ASW_ShaftControl/1(Shaft1GearReq)
  [Fork3DeltaSpdReq] -> ASW_GearPressureControl/15(Fork3DeltaSpdReq)
  [EngTqVal] -> ASW_ClutchControl_new/6(EngTq)
  ASW_Interface/22(MaiLineSolnIVal) -> [MaiLineSolnIVal]
  ASW_Interface/12(Fork2PosnVal) -> [Fork2PosnVal]
  [AccPedlCanVal] -> ASW_Interface/1(AccPedlCanVal)
  ASW_ShaftControl/7(Shaft1GearErr) -> Terminator3/1
  ASW_ClutchPressureControl/4(CluSoln2IReq) -> [CluSoln2IReq]
  ASW_GearPositioner/19(Fork4DirReq) -> [Fork4DirReq]
  [Fncall_ShaftCtrl] -> ASW_ShaftControl/Trigger
  ASW_ShaftAccessControl/7(TrsmNrGearErr) -> Terminator/1
  ASW_ClutchControl_new/2(Clu2Act) -> [Clu2Act]
  [Fork2DeltaSpdAct] -> ASW_GearPressureControl/11(Fork2DeltaSpdAct)
  [Fork1PosnReq] -> ASW_GearPressureControl/4(Fork1PosnReq)
  [EngSpdCanVal] -> ASW_Interface/25(EngSpdCanVal)
  ASW_Interface/10(VehSpdTrsmEstimd) -> [VehSpdTrsmEstimd]
  [VehSpdCanVal] -> ASW_Interface/4(VehSpdCanVal)
  [Shaft2GearAct] -> ASW_ShaftAccessControl/4("Shaft2GearAct ")
  [Shaft2GearReq] -> ASW_ShaftControl/2(Shaft2GearReq)
  [Clu1PReqFlg] -> Terminator5/1
  [EngSpdVal] -> Terminator4/1
  [CluSoln2IRawVal] -> ASW_Interface/23(CluSoln2IRawVal)
  [SolnOutpTVal] -> ASW_GearPressureControl/26(SolnOutpTVal)

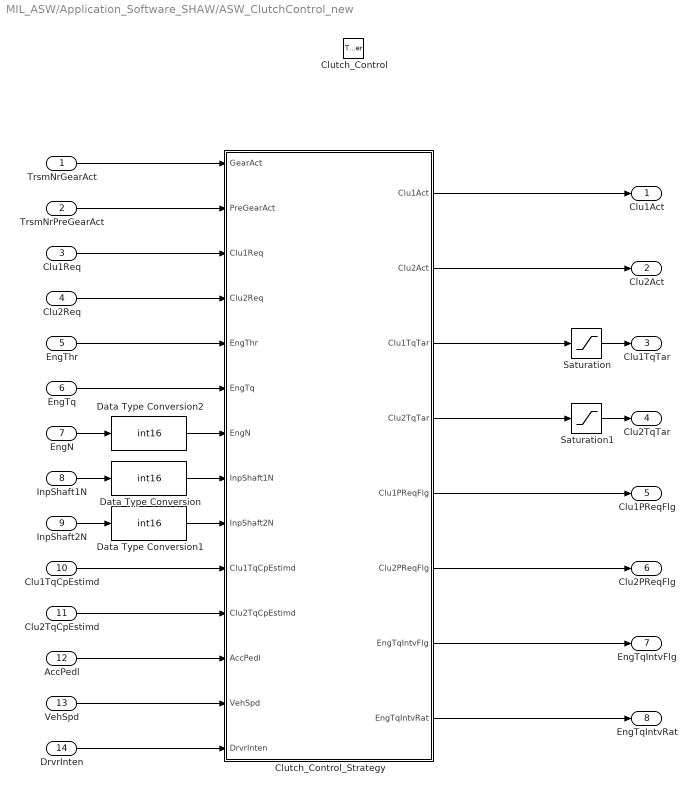
== system MIL_ASW/Application_Software_SHAW/ASW_ClutchControl_new ==
  TrsmNrGearAct : Inport
  TrsmNrPreGearAct : Inport  Port=2
  Clu1Req : Inport  Port=3
  Clu2Req : Inport  Port=4
  EngThr : Inport  Port=5
  EngTq : Inport  Port=6
  EngN : Inport  Port=7
  InpShaft1N : Inport  Port=8
  InpShaft2N : Inport  Port=9
  Clu1TqCpEstimd : Inport  Port=10
  Clu2TqCpEstimd : Inport  Port=11
  AccPedl : Inport  Port=12
  VehSpd : Inport  Port=13
  DrvrInten : Inport  Port=14
  Clutch_Control : TriggerPort  TriggerType=function-call  VariantControl=(inherit)  PortDimensions=1
  Clutch_Control_Strategy : Stateflow chart  TreatAsAtomicUnit=on
  Data Type Conversion : DataTypeConversion  OutDataTypeStr=int16
  Data Type Conversion1 : DataTypeConversion  OutDataTypeStr=int16
  Data Type Conversion2 : DataTypeConversion  OutDataTypeStr=int16
  Saturation : Saturate  UpperLimit=EngTqMaxNorm  LowerLimit=0  OutDataTypeStr=uint16
  Saturation1 : Saturate  UpperLimit=EngTqMaxNorm  LowerLimit=0  OutDataTypeStr=uint16
  Clu1Act : Outport  VectorParamsAs1DForOutWhenUnconnected=off
  Clu2Act : Outport  Port=2  VectorParamsAs1DForOutWhenUnconnected=off
  Clu1TqTar : Outport  Port=3  VectorParamsAs1DForOutWhenUnconnected=off
  Clu2TqTar : Outport  Port=4  VectorParamsAs1DForOutWhenUnconnected=off
  Clu1PReqFlg : Outport  Port=5  VectorParamsAs1DForOutWhenUnconnected=off
  Clu2PReqFlg : Outport  Port=6  VectorParamsAs1DForOutWhenUnconnected=off
  EngTqIntvFlg : Outport  Port=7  VectorParamsAs1DForOutWhenUnconnected=off
  EngTqIntvRat : Outport  Port=8  VectorParamsAs1DForOutWhenUnconnected=off
  wires:
  Saturation1/1 -> Clu2TqTar/1
  Saturation/1 -> Clu1TqTar/1
  Clutch_Control_Strategy/1(Clu1Act) -> Clu1Act/1
  Clutch_Control_Strategy/2(Clu2Act) -> Clu2Act/1
  TrsmNrGearAct/1 -> Clutch_Control_Strategy/1(GearAct)
  TrsmNrPreGearAct/1 -> Clutch_Control_Strategy/2(PreGearAct)
  Clu1Req/1 -> Clutch_Control_Strategy/3(Clu1Req)
  Clu2Req/1 -> Clutch_Control_Strategy/4(Clu2Req)
  EngThr/1 -> Clutch_Control_Strategy/5(EngThr)
  EngN/1 -> Data Type Conversion2/1
  InpShaft1N/1 -> Data Type Conversion/1
  InpShaft2N/1 -> Data Type Conversion1/1
  AccPedl/1 -> Clutch_Control_Strategy/12(AccPedl)
  VehSpd/1 -> Clutch_Control_Strategy/13(VehSpd)
  Clutch_Control_Strategy/7(EngTqIntvFlg) -> EngTqIntvFlg/1
  Clutch_Control_Strategy/8(EngTqIntvRat) -> EngTqIntvRat/1
  Clutch_Control_Strategy/5(Clu1PReqFlg) -> Clu1PReqFlg/1
  Clutch_Control_Strategy/6(Clu2PReqFlg) -> Clu2PReqFlg/1
  Data Type Conversion/1 -> Clutch_Control_Strategy/8(InpShaft1N)
  Data Type Conversion1/1 -> Clutch_Control_Strategy/9(InpShaft2N)
  Data Type Conversion2/1 -> Clutch_Control_Strategy/7(EngN)
  DrvrInten/1 -> Clutch_Control_Strategy/14(DrvrInten)
  Clu1TqCpEstimd/1 -> Clutch_Control_Strategy/10(Clu1TqCpEstimd)
  Clu2TqCpEstimd/1 -> Clutch_Control_Strategy/11(Clu2TqCpEstimd)
  Clutch_Control_Strategy/3(Clu1TqTar) -> Saturation/1
  Clutch_Control_Strategy/4(Clu2TqTar) -> Saturation1/1
  EngTq/1 -> Clutch_Control_Strategy/6(EngTq)

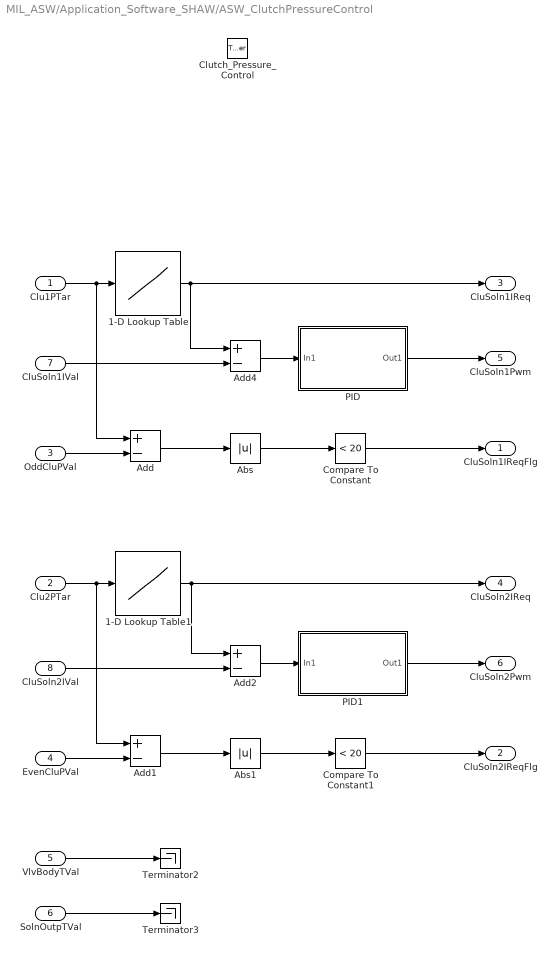
== system MIL_ASW/Application_Software_SHAW/ASW_ClutchPressureControl ==
  Clu1PTar : Inport
  Clu2PTar : Inport  Port=2
  OddCluPVal : Inport  Port=3
  EvenCluPVal : Inport  Port=4
  VlvBodyTVal : Inport  Port=5
  SolnOutpTVal : Inport  Port=6
  CluSoln1IVal : Inport  Port=7
  CluSoln2IVal : Inport  Port=8
  Clutch_Pressure_Control : TriggerPort  TriggerType=function-call  VariantControl=(inherit)  PortDimensions=1
  1-D Lookup Table : Lookup_n-D  NumberOfTableDimensions=1  BreakpointsForDimension1=CluSoln1LineP  BreakpointsForDimension1DataTypeStr=Inherit: Inherit from 'Breakpoint data'  Table=CluSoln1LineI  TableDataTypeStr=Inherit: Inherit from 'Table data'  ExtrapMethod=Clip  UseLastTableValue=on  InternalRulePriority=Speed  OutDataTypeStr=Inherit: Inherit from 'Table data'  RndMeth=Simplest  InputSameDT=on
  1-D Lookup Table1 : Lookup_n-D  NumberOfTableDimensions=1  BreakpointsForDimension1=CluSoln2LineP  BreakpointsForDimension1DataTypeStr=Inherit: Inherit from 'Breakpoint data'  Table=CluSoln2LineI  TableDataTypeStr=Inherit: Inherit from 'Table data'  ExtrapMethod=Clip  UseLastTableValue=on  InternalRulePriority=Speed  OutDataTypeStr=Inherit: Inherit from 'Table data'  RndMeth=Simplest  InputSameDT=on
  Abs : Abs  OutDataTypeStr=uint16
  Abs1 : Abs  OutDataTypeStr=uint16
  Add{,1..2,4} (4 alike) : Sum  Inputs=+-  OutDataTypeStr=int16
  Compare To Constant : simulink/Logic and Bit Operations/Compare To Constant  relop=<  const=20  OutDataTypeStr=uint8
  Compare To Constant1 : simulink/Logic and Bit Operations/Compare To Constant  relop=<  const=20  OutDataTypeStr=uint8
  PID : Subsystem
  PID1 : Subsystem
  Terminator2 : Terminator
  Terminator3 : Terminator
  CluSoln1IReqFlg : Outport  VectorParamsAs1DForOutWhenUnconnected=off
  CluSoln2IReqFlg : Outport  Port=2  VectorParamsAs1DForOutWhenUnconnected=off
  CluSoln1IReq : Outport  Port=3  VectorParamsAs1DForOutWhenUnconnected=off
  CluSoln2IReq : Outport  Port=4  VectorParamsAs1DForOutWhenUnconnected=off
  CluSoln1Pwm : Outport  Port=5  VectorParamsAs1DForOutWhenUnconnected=off
  CluSoln2Pwm : Outport  Port=6  VectorParamsAs1DForOutWhenUnconnected=off
  wires:
  Clu1PTar/1 -> Add/1, 1-D Lookup Table/1
  Add/1 -> Abs/1
  Compare To Constant/1 -> CluSoln1IReqFlg/1
  VlvBodyTVal/1 -> Terminator2/1
  SolnOutpTVal/1 -> Terminator3/1
  1-D Lookup Table/1 -> CluSoln1IReq/1, Add4/1
  Abs/1 -> Compare To Constant/1
  OddCluPVal/1 -> Add/2
  Clu2PTar/1 -> Add1/1, 1-D Lookup Table1/1
  Add1/1 -> Abs1/1
  Compare To Constant1/1 -> CluSoln2IReqFlg/1
  Abs1/1 -> Compare To Constant1/1
  EvenCluPVal/1 -> Add1/2
  CluSoln1IVal/1 -> Add4/2
  Add4/1 -> PID/1(In1)
  PID/1(Out1) -> CluSoln1Pwm/1
  1-D Lookup Table1/1 -> CluSoln2IReq/1, Add2/1
  CluSoln2IVal/1 -> Add2/2
  Add2/1 -> PID1/1(In1)
  PID1/1(Out1) -> CluSoln2Pwm/1

== system MIL_ASW/Application_Software_SHAW/ASW_DrivingStrategy ==
  SftLvrVal : Inport
  AccPedlVal : Inport  Port=2
  BrkPedlVal : Inport  Port=3
  BrkSig : Inport  Port=4
  CrnkSpdVal : Inport  Port=5
  VehSpdVal : Inport  Port=6
  TrsmNrPreGearAct : Inport  Port=7
  TrsmNrGearAct : Inport  Port=8
  Driving_Strategy : TriggerPort  TriggerType=function-call  VariantControl=(inherit)  PortDimensions=1
  Auto_Mode_Decision : Subsystem  TreatAsAtomicUnit=on
  Bus Creator : BusCreator  Inputs=8
  Bus Selector : BusSelector  OutputSignals=SftLvrVal
  Bus Selector1 : BusSelector  OutputSignals=SftLvrVal,AccPedlVal,BrkPedlVal,BrkSig,VehSpdVal,CrnkSpdVal,TrsmNrGearAct,TrsmNrPreGearAct
  Bus Selector2 : BusSelector  OutputSignals=AccPedlVal
  Driver_Detection : Subsystem
  Fast_Off_Detection : Subsystem  Commented=on
  Load_Detection : Subsystem  Commented=on
  Manual_Mode_Decision : Subsystem  Commented=on
  Road_Detection : Subsystem  Commented=on
  Synthesis_Check : Subsystem  TreatAsAtomicUnit=on
  TrsmNrPreGearReq : Outport  VectorParamsAs1DForOutWhenUnconnected=off
  TrsmNrGearReq : Outport  Port=2  VectorParamsAs1DForOutWhenUnconnected=off
  DrvrInten : Outport  Port=3  VectorParamsAs1DForOutWhenUnconnected=off
  wires:
  SftLvrVal/1 -> Bus Creator/1  "SftLvrVal"
  AccPedlVal/1 -> Bus Creator/2  "AccPedlVal"
  BrkPedlVal/1 -> Bus Creator/3  "BrkPedlVal"
  VehSpdVal/1 -> Bus Creator/6  "VehSpdVal"
  TrsmNrPreGearAct/1 -> Bus Creator/7  "TrsmNrPreGearAct"
  TrsmNrGearAct/1 -> Bus Creator/8  "TrsmNrGearAct"
  Synthesis_Check/1(TrsmNrPreGearReq) -> TrsmNrPreGearReq/1
  Synthesis_Check/2(TrsmNrGearReq) -> TrsmNrGearReq/1
  Bus Selector1/1 -> Auto_Mode_Decision/1(SftLvrVal)  "<SftLvrVal>"
  Bus Selector1/2 -> Auto_Mode_Decision/2(AccPedlVal)  "<AccPedlVal>"
  Bus Selector1/3 -> Auto_Mode_Decision/3(BrkVal)  "<BrkPedlVal>"
  Bus Selector1/5 -> Auto_Mode_Decision/5(VehSpdVal)  "<VehSpdVal>"
  Bus Selector1/6 -> Auto_Mode_Decision/6(CrnkSpdVal)  "<CrnkSpdVal>"
  Bus Selector1/7 -> Auto_Mode_Decision/7(TrsmNrGearAct)  "<TrsmNrGearAct>"
  Bus Selector1/8 -> Auto_Mode_Decision/8(TrsmNrPreGearAct)  "<TrsmNrPreGearAct>"
  Auto_Mode_Decision/1(TrsmNrPreGearTarAutMod) -> Synthesis_Check/2(TrsmNrPreGearTarAutMod)
  Auto_Mode_Decision/2(TrsmNrGearTarAutMod) -> Synthesis_Check/3(TrsmNrGearTarAutMod)
  CrnkSpdVal/1 -> Bus Creator/5  "CrnkSpdVal"
  Bus Selector/1 -> Synthesis_Check/1(SftLvrVal)  "<SftLvrVal>"
  BrkSig/1 -> Bus Creator/4  "BrkSig"
  Bus Selector1/4 -> Auto_Mode_Decision/4(BrkSig)  "<BrkSig>"
  Driver_Detection/1(Inten) -> Auto_Mode_Decision/9(DrvrInten), DrvrInten/1
  Bus Creator/1 -> Bus Selector/1, Bus Selector1/1, Bus Selector2/1
  Bus Selector2/1 -> Driver_Detection/1(AccPedl)  "<AccPedlVal>"
